simulink model "Function5"  (R2020a)
settings: Solver=FixedStepDiscrete  StartTime=0.0  StopTime=0.1  FixedStep=0.1  RelTol=1e-3  EnableMultiTasking=on
settings Model: Creator=bzhan  LastModifiedBy=bzhan
settings SolverCC: AutoInsertRateTranBlk=on
settings DataIOCC: LimitDataPoints=on
settings OptimizationCC: LifeSpan=inf
settings DebuggingCC: AllowSymbolicDim=off  SFUnexpectedBacktrackingDiag=warning  SFNoUnconditionalDefaultTransitionDiag=warning  SFExecutionAtInitializationDiag=none  ArithmeticOperatorsInVariantConditions=warning
settings SFSimCC: SimUseLocalCustomCode=off  CustomCodeUndefinedFunction=UseInterfaceOnly
settings RTWCC: RTWUseLocalCustomCode=off
settings CodeAppCC: StateflowObjectComments=on
settings GRTTargetCC: TargetLangStandard=C89/C90 (ANSI)
settings ConfigComp: CovMetricSettings=dw  CovHtmlReporting=on  CovSaveCumulativeToWorkspaceVar=on  CovSaveSingleToWorkspaceVar=on  CovShowResultsExplorer=off  CovExternalEMLEnable=off  CovSFcnEnable=off

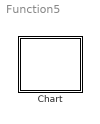
== system Function5 ==
  Chart : Stateflow chart  TreatAsAtomicUnit=on

== stateflow chart Function5/Chart ==
  state A
    en: f("en_A")
  state B
    en: f("en_B")
  (default) -> A : {b=[0 1;2 3];}
  (junction 29) -> B : [b(1,1)==3 && b(1,2)==1]
  A -> (junction 29) : {compute()}
  data: s function_input; b local double size=2 2 =[0 0;0 0]
  function compute:
    | function compute
    |   if b(1,1) < b(2,2)
    |     b(1,1)=b(2,2);
    |   end
    |   if b(2,1) < b(1,2)
    |     b(2,1)=b(1,2);
    |   end
  function f(s):
    | function f(s)
    |   fprintf(s+"\n");
